simulink model "modelref_base"  (R2022a)
settings: Solver=FixedStepDiscrete  StartTime=0.0  StopTime=10.0  RelTol=1e-3  EnableMultiTasking=on
InitFcn:
  | mbd_cmd_check;
model workspace (MAT data in the model file):
  modelws_data = 3
undefined symbols (not defined in the file or in its folder): data
settings Model: DataDictionary=modelref.sldd  Creator=KenYoshioka  LastModifiedBy=KenYoshioka
settings SolverCC: AutoInsertRateTranBlk=on
settings OptimizationCC: DefaultParameterBehavior=Inlined  DefaultUnderspecifiedDataType=single  EnhancedBackFolding=on  PassReuseOutputArgsAs=Individual arguments  ZeroExternalMemoryAtStartup=off  ZeroInternalMemoryAtStartup=off  OptimizeBlockOrder=speed  DifferentSizesBufferReuse=on  OptimizationCustomize=off  EfficientTunableParamExpr=on
settings DebuggingCC: ParameterTunabilityLossMsg=error
settings HardwareCC: ProdBitPerPointer=32  ProdBitPerSizeT=32  ProdBitPerPtrDiffT=32  ProdLargestAtomicInteger=Long  ProdLargestAtomicFloat=Double  ProdWordSize=32  ProdHWDeviceType=ARM Compatible->ARM Cortex
settings ModelReferenceCC: ModelReferenceNumInstancesAllowed=Single
settings SFSimCC: MATLABDynamicMemAlloc=off
settings RTWCC: SystemTargetFile=ert.tlc  GenCodeOnly=on  TemplateMakefile=ert_default_tmf  Toolchain=GNU Tools for ARM Embedded Processors
settings CodeAppCC: ForceParamTrailComments=on  IgnoreCustomStorageClasses=off  MaxIdLength=255  OperatorAnnotations=on  SimulinkDataObjDesc=on  SFDataObjDesc=on  InsertBlockDesc=on
settings ERTTargetCC: GenerateSampleERTMain=on  InlinedParameterPlacement=NonHierarchical  ERTCustomFileTemplate=example_file_process.tlc

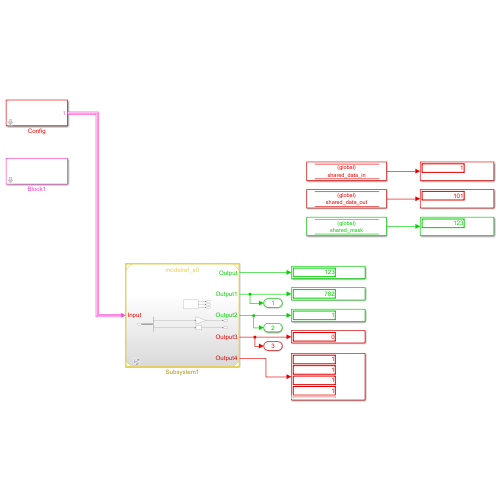
[thumbnail: Simulink's stored preview of the top-level diagram]
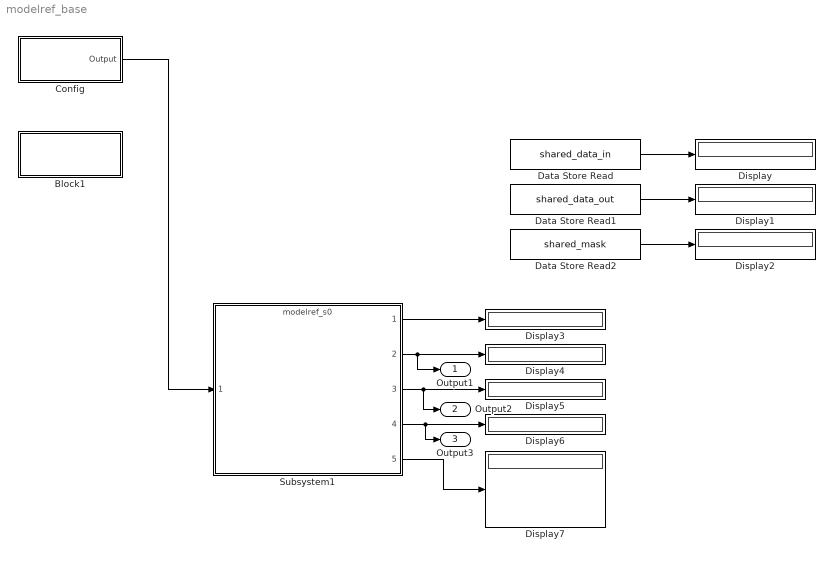
== system modelref_base ==
  Block1 : Subsystem
      mask init:
      | evalin('base','mbd_diag = Mbd_diag.instance();')
      | Local = evalin('base','mbd_diag;');
      | 
      | %Local_entry_shared_index = getEntry(Local.ddSec,'shared_index');
      | %Local_param_shared_index = getValue(Local_entry_shared_index);
      | global Global_signal_index;
      | global Global_local_index;
      | if (~Local.portalSignalInit)
      |     disp('Global_signal_index clear');
      |     Global_signal_index = 0;
      |     Global_local_index = 0;
      | 
      | %    Local_param_shared_index.Value = 0;
      | %    setValue(Local_entry_shared_index, Local_param_shared_index);
      | end
      | Global_signal_index = Global_signal_index + 1;
      | Global_local_index = Global_local_index + 1;
      | Local.portalSignalInit = 1;
      | 
      | %Local_param_shared_index.Value = Local_param_shared_index.Value + 1;
      | %setValue(Local_entry_shared_index, Local_param_shared_index);
      | 
      | %assignin('base', 'mbd_diag_temp', Local);
      | %evalin('base', 'mbd_diag = mbd_diag_temp;');
  Config : Subsystem
      mask init:
      | global Mask_shared_data;
      | Mask_shared_data = uint32(123);
      | 
      | global Global_local_index;
      | Global_local_index = 0;
      | 
      | global Global_array;
      | Global_array = zeros(1,100,'uint8');
      | 
      | mws = get_param(bdroot(gcb),'ModelWorkspace');
      | disp('base');
      | disp(mws.getVariable('modelws_data'));
  Data Store Read : DataStoreRead  DataStoreName=shared_data_in  SampleTime=0.001  IndexOptions=Index vector (dialog)  Indices=1  OutputSizes=1
  Data Store Read1 : DataStoreRead  DataStoreName=shared_data_out  SampleTime=0.001  IndexOptions=Index vector (dialog)  Indices=1  OutputSizes=1
  Data Store Read2 : DataStoreRead  DataStoreName=shared_mask  SampleTime=0.01  IndexOptions=Index vector (dialog)  Indices=1  OutputSizes=1
  Display{,1..7} (8 alike) : Display
  Subsystem1 : ModelReference  ModelNameDialog=modelref_s0  SimulationMode=Normal  ModelReferenceVersion=1.46
  Output1 : Outport
  Output2 : Outport  Port=2
  Output3 : Outport  Port=3
  wires:
  Data Store Read/1 -> Display/1
  Data Store Read1/1 -> Display1/1
  Data Store Read2/1 -> Display2/1
  Subsystem1/1 -> Display3/1
  Subsystem1/2 -> Display4/1, Output1/1
  Subsystem1/3 -> Display5/1, Output2/1
  Subsystem1/4 -> Display6/1, Output3/1
  Subsystem1/5 -> Display7/1
  Config/1(Output) -> Subsystem1/1

== system modelref_base/Block1 ==

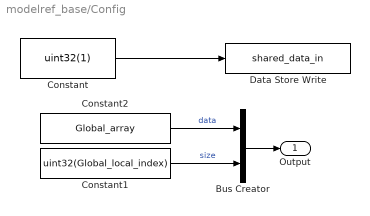
== system modelref_base/Config ==
  Bus Creator : BusCreator  Inputs=data,size  OutDataTypeStr=Bus: shared_bus_t
  Constant : Constant  Value=uint32(1)  SampleTime=0.001
  Constant1 : Constant  Value=uint32(Global_local_index)
  Constant2 : Constant  Value=Global_array
  Data Store Write : DataStoreWrite  DataStoreName=shared_data_in  IndexOptions=Index vector (dialog)  Indices=1  OutputSizes=1
  Output : Outport
  wires:
  Constant/1 -> Data Store Write/1
  Constant1/1 -> Bus Creator/2  "size"
  Constant2/1 -> Bus Creator/1  "data"
  Bus Creator/1 -> Output/1
